simulink model "Cruise_Model_V8_QRTuning_TFLim"  (R2024a)
settings: Solver=ode23t  StartTime=0.0  StopTime=20  RelTol=1e-3
values from neighbouring files (symbols this model uses):
  F = fullfile(P,S(k).name)    [extractNACAdata.m]
  mission = struct()    [runMission.m]
  r = fuselage(i).diameter/2    [plotConfiguration.m]
  referenceGeo =     [alexisignoringme.mat]    (also in testing.mat)
undefined symbols (not defined in the file or in its folder): coefficients, dir, K, kb, kt, Light, MIL, Ue, Xe, Xes, xyz_tr
libraries: slpidlib x14, aerolibwind2 x8, aerolibatmos2 x4, shared6dof x1
(part 3 of 3)

== system Cruise_Model_V8_QRTuning_TFLim/Trim Solver and Actuation/Controller/PID_GBDP_withThrust/Subsystem/Step demand for testing1 ==
  Va : Inport
  Mux1 : Mux  Inputs=2
  Scope2 : Scope
  Scope4 : Scope
  Step1 : Step  Time=60  Before=25  After=31  SampleTime=0
  Step2 : Step  Time=80  After=-3  SampleTime=0
  Step3 : Step  Time=120  After=-5  SampleTime=0
  Step4 : Step  Time=100  After=8  SampleTime=0
  Step5 : Step  Time=140  After=-2  SampleTime=0
  Sum : Sum  Inputs=+++++
  To Workspace : ToWorkspace  VariableName=airspeedResponse  SaveFormat=Timeseries  SampleTime=-1
  Out1 : Outport
  wires:
  Step2/1 -> Sum/2
  Va/1 -> Scope2/1, Mux1/2
  Step1/1 -> Sum/1
  Step4/1 -> Sum/4
  Sum/1 -> Mux1/1, Out1/1
  Mux1/1 -> Scope4/1, To Workspace/1
  Step3/1 -> Sum/3
  Step5/1 -> Sum/5

== matlab function Cruise_Model_V8_QRTuning_TFLim/Trim Solver and Actuation/Controller/Trim Solver/Stop Time (Real)/MATLAB Function ==
  data: y output
function y = fcn()
%#codegen

persistent t0
coder.extrinsic('cputime');

if isempty(t0)
    y = 0;
    t0 = 0;
    t0 = cputime;
end

y = cputime;
y = y-t0;

== matlab function Cruise_Model_V8_QRTuning_TFLim/Aircraft Dynamics/Aerodynamic Forces and Moments/MATLAB Function ==
  data: Fb output; Mcg output; coeff input Bus: coeff; u input; alpha input; beta input; V input; rho input; X input; refGeo parameter; m parameter; thrust input; cg parameter
function [Fb,Mcg] = aeroDyn(coeff, u, alpha, beta, V, rho, X, refGeo, m, thrust, cg)
% Function aeroDyn simulates ....

%% Setting up intermediate variables
b = refGeo.bref;
S = refGeo.Sref;
c = refGeo.cref;

Q = 0.5*rho*V^2; % Dynamic pressure Q

ndc = c/(2*V);
ndb = b/(2*V);

%% Seperating vectors (BFR)
uvw = X(1:3); % Translational velocity vector
pqr = X(4:6); % Angular velocity vector
EA = X(7:end);

%% Handle Stall

%% Non-dimensional Aerodynamic Force Coefficients
% In wind axis
% Lift
CL = applyDeriv(coeff.CL0, coeff.CLa, coeff.CLb, coeff.CLn, 0, coeff.CLq, 0, u, alpha, beta, pqr, ndc);

% Drag 
CD = applyDeriv(coeff.CD0, coeff.CDa, coeff.CDb, coeff.CDn, 0, 0, 0, u, alpha, beta, pqr, ndc);

% Sideforce
CY = applyDeriv(0, coeff.CYa, coeff.CYb, coeff.CYn, coeff.CYp, 0, coeff.CYr, u, alpha, beta, pqr, ndb);

if abs(alpha) > 14.5*(pi/180)
    CL = 0;
    CD = coeff.CD0;
end

%% Rotate wind to body
Faw = [-max(CD,0); CY; -CL].*Q*S; % Force vector in the stability frame

Rwb = [cos(alpha)*cos(beta), -cos(alpha)*sin(beta), -sin(alpha);  
       sin(beta)           ,  cos(beta)           ,  0         ; 
       cos(beta)*sin(alpha), -sin(alpha)*sin(beta),  cos(alpha)];

Fab = Rwb*Faw; % aerodynamic force on body

%% Aerodynamic Moment about CG
% In Fb, with moments taken about the centre of gravity

% Roll
Cl = applyDeriv(0, coeff.Cla, coeff.Clb, coeff.Cln, coeff.Clp, 0, coeff.Clr, u, alpha, beta, pqr, ndb);

% Pitch
Cm = applyDeriv(coeff.Cm0, coeff.Cma, coeff.Cmb, coeff.Cmn, 0, coeff.Cmq, 0, u, alpha, beta, pqr, ndc);

% Yaw
Cn = applyDeriv(0, coeff.Cna, coeff.Cnb, coeff.Cnn, coeff.Cnp, 0, coeff.Cnr, u, alpha, beta, pqr, ndb);

if abs(alpha) > 20*(pi/180)
    Cm = 0;
end

Ma = [b*Cl; c*Cm; b*Cn].*Q*S;

%% Propulsion Effects
% Moment and forces induced by throttle
FTb = zeros(3, length(thrust.Tinit));
MTcg = zeros(3, length(thrust.Tinit));

FTb = zeros(3, length(thrust.Tinit));
MTcg = zeros(3, length(thrust.Tinit));

for i = 1:length(thrust.Tinit)
    kt = thrust.kt(i,:);
    kb = thrust.kb(i,:);
    dir = thrust.dir(i,:);

    idx = length(coeff.CLn) + 1 + (i-1)*4; % index of thrust-deflection pairs for thrust objects
    FTt = [0      ; % Thrust in rotor plane
           0      ;
           -kt*u(idx)^2];

    MTy = [0      ;
           0      ;
           dir*kb*(u(idx)^2)];
    
    Rrb = transMatrix([u(idx+1) u(idx+2) u(idx+3)].*[1 1 1]); % rotation matrix from rotor plane to body, first converting to geometric axis

    FTb(:,i) = Rrb*FTt; % Rotate to body frame, switching from geometric to dynamic coordinates
    MTcg(:,i) = Rrb*MTy + cross(thrust.xyz_tr(i,:) - cg, FTb(:,i))';
end

FTb = sum(FTb,2);
MTcg = sum(MTcg,2);

% Gravity Effects
Fgb = [-9.81*sin(X(8))          ; % Body frame
        9.81*cos(X(8))*sin(X(7));
        9.81*cos(X(8))*cos(X(7))]*m; % ASSUMPTION: Constant Mass

%% Out
Rbe = body2earth(X(7), X(8), X(9));

Fb = FTb + Fgb + Fab;
Mcg = MTcg + Ma;

forces = [FTb; Fgb; Fab; Rbe*Fb];
aero = [CL; CD; Cm];
uvw_e = Rbe*X(1:3);

end

%% Extra functions

function C = applyDeriv(C0, Ca, Cb, Cn, Cp, Cq, Cr, u, alpha, beta, pqr, nd)
% function applyDeriv calculates the coefficient C from the derivatives C0,
% Ca, Cb, Cn wrt 0, alpha, beta and control (n), respectively.

    C_nc = C0 + Ca*alpha + Cb*beta + Cp*pqr(1)*nd + Cq*pqr(2)*nd + Cr*pqr(3)*nd; % lift coefficient no control
    
    C_c = (Cn.*u(1:length(Cn)))';

    C = C_nc + sum(C_c);

end

== matlab function Cruise_Model_V8_QRTuning_TFLim/Trim Solver and Actuation/Controller/Trim Solver/MATLAB Function ==
  data: u input; U output; kb input; kt input; dir input; xyz_tr input; Ue input
function U = fcn(u, kb, kt, dir, xyz_tr, Ue)

nT = 4;
nc = 3;

thrust = struct();
thrust.kb = kb;
thrust.kt = kt;
thrust.dir = dir;
thrust.Tinit = [0 0 0 0];
thrust.xyz_tr = xyz_tr;

Ur = torqueForce2U(u(4:6), u(1:3), thrust, Ue, nc, nT, 150, [1.1 0 0]);
U = [u(1:3)' Ur(1) 0 0 0 Ur(2) 0 0 0 Ur(3) 0 0 0 Ur(4) 0 0 0]';
